simulink model "FBsimDC"  (R2018b)
settings: Solver=ode4  StartTime=0.0  StopTime=0.5e-3*1+0.05*0  FixedStep=Tsim  MaxStep=1e-4  RelTol=1e-6
undefined symbols (not defined in the file): fsw, J, Kt, La, Ra, sigbuilder_block, Ts, Vdc
libraries: powerlib x9, simulink x4, powerlib_meascontrol x1
settings Model: Creator=Mattia  LastModifiedBy=matti
settings DataIOCC: ReturnWorkspaceOutputs=on

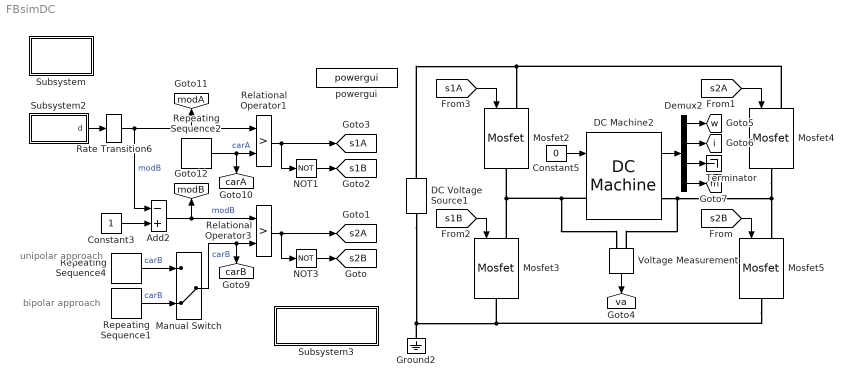
== system FBsimDC ==
  note: unipolar approach
  note: bipolar approach
  Add2 : Sum  Inputs=-+
  Constant3 : Constant  SampleTime=1/(200*fsw)*0+Ts
  Constant5 : Constant  Value=0  SampleTime=1/(200*fsw)
  DC Machine2 : powerlib/Machines/DC Machine  PresetModel=No  MechanicalLoad=Torque TL  FieldType=Permanent magnet  ShowDetailedParameters=on  MeasurementBus=off  RLa="[Ra  La]"  RLf="[ 240  120]"  Laf=1.8  MachineConstant=Torque constant (N.m/A)  Ke=1.8  Kt=Kt  J=J  Bm=B  Tf=0  w0=0  Ifinit=1  TsPowergui=0  TsBlock=-1
      settings: SourceProductName=Simscape Electrical
  DC Voltage Source1 : powerlib/Electrical Sources/DC Voltage Source  Amplitude=Vdc  Measurements=None
      settings: SourceProductName=Simscape Electrical
  Demux2 : Demux  BusSelectionMode=on
  Ground2 : powerlib/Elements/Ground  LConnTagsString=a
      settings: SourceProductName=Simscape Electrical
  Manual Switch : ManualSwitch  CurrentSetting=0
  Mosfet{2..5} (4 alike) : powerlib/Power Electronics/Mosfet  Ron=0.1  Lon=0  Rd=0.01  Vfd=0  IC=0  Rs=1e5  Cs=inf  Measurements=off
      settings: SourceProductName=Simscape Electrical
  NOT1 : Logic  Operator=NOT  IconShape=distinctive  AllPortsSameDT=off  OutDataTypeStr=boolean
  NOT3 : Logic  Operator=NOT  IconShape=distinctive  AllPortsSameDT=off  OutDataTypeStr=boolean
  Rate Transition6 : RateTransition  OutPortSampleTime=Ts
  Relational Operator1 : RelationalOperator  Operator=>  OutDataTypeStr=boolean  RndMeth=Simplest
  Relational Operator3 : RelationalOperator  Operator=>  OutDataTypeStr=boolean  RndMeth=Simplest
  Repeating Sequence1 : simulink/Sources/Repeating Sequence  rep_seq_t=[0 1/(2*fsw) 1/fsw]  rep_seq_y=[1 0 1]
  Repeating Sequence2 : simulink/Sources/Repeating Sequence  rep_seq_t=[0 1/(2*fsw) 1/fsw]  rep_seq_y=[0 1 0]
  Repeating Sequence4 : simulink/Sources/Repeating Sequence  rep_seq_t=[0 1/(2*fsw) 1/fsw]  rep_seq_y=[0 1 0]
  Subsystem : Subsystem
      mask Display: disp('stream')
  Subsystem2 : Subsystem
      mask Display: disp('reference')
  Subsystem3 : Subsystem
      mask Display: disp('embedded version')
  Terminator : Terminator
  Voltage Measurement : powerlib/Measurements/Voltage Measurement  PhasorSimulation=off  OutputType=Complex  PSBequivalent=0
  powergui : powerlib/powergui  Priority=1  SimulationMode=Continuous  SampleTime=1/(400*fsw)  frequency=60  Iterations=50  frequencyindice=0  Pbase=100e6  ErrMax=1e-4  UnitsV=kV  UnitsW=MW  buscounter=0  FunctionMessages=off  echomessages=off  EnableUseOfTLC=off  CurrentSourceSwitches=off  DisableSnubberDevices=on  DisableRonSwitches=on  DisableVfSwitches=on  DisplayEquations=off  SolverType=Tustin/Backward Euler (TBE)  Interpol=off  ExternalGateDelay=off  methode=off  Ts=100  x0status=blocks  SPID=off  SwTol=0  HookPort=off  RestoreLinks=warning  ResistiveCurrentMeasurement=off  Frange=[0:2:500]  Ylog=off  Xlog=on  ShowGrid=off  save=off  variable=ZData  structure=0  ZoomFFT=off  StartTime=0.0  cycles=1  DisplayStyle=1  fundamental=60  FreqAxis=off  MaxFrequency=1000  frequencyindicesteady=1  RmsSteady=1  display=off
  tag scope: carA=global, carB=global, i=global, m=global, modA=global, modB=global, s1A=global, s1B=global, s2A=global, s2B=global, va=global, w=global
  wires:
  NOT1/1 -> [s1B]
  DC Machine2/1 -> Demux2/1
  [s2B] -> Mosfet5/1
  [s2A] -> Mosfet4/1
  [s1B] -> Mosfet3/1
  [s1A] -> Mosfet2/1
  Demux2/3 -> Terminator/1
  Voltage Measurement/1 -> [va]
  Manual Switch/1 -> [carB], Relational Operator3/2  "carB"
  NOT3/1 -> [s2B]
  Repeating Sequence2/1 -> [carA], Relational Operator1/2  "carA"
  Subsystem2/1(d) -> Rate Transition6/1
  Constant3/1 -> Add2/2
  Repeating Sequence4/1 -> Manual Switch/1  "carB"
  Rate Transition6/1 -> Add2/1, Relational Operator1/1, [modA]  "modB"
  Repeating Sequence1/1 -> Manual Switch/2  "carB"
  Constant5/1 -> DC Machine2/1
  Demux2/1 -> [w]
  Demux2/2 -> [i]
  Demux2/4 -> [m]
  Add2/1 -> [modB], Relational Operator3/1  "modB"
  Relational Operator3/1 -> [s2A], NOT3/1
  Relational Operator1/1 -> NOT1/1, [s1A]
  connections:
  Mosfet3/RConn1 -- Mosfet5/RConn1 -- Ground2/LConn1 -- DC Voltage Source1/LConn1
  Mosfet4/LConn1 -- DC Voltage Source1/RConn1 -- Mosfet2/LConn1
  Mosfet4/RConn1 -- Voltage Measurement/LConn2 -- DC Machine2/RConn1 -- Mosfet5/LConn1
  Mosfet3/LConn1 -- Voltage Measurement/LConn1 -- DC Machine2/LConn1 -- Mosfet2/RConn1

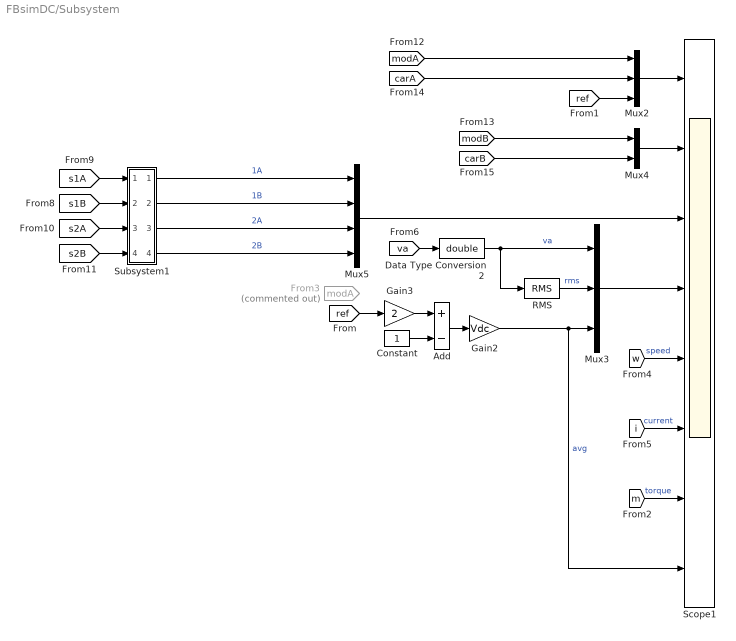
== system FBsimDC/Subsystem ==
  Add : Sum  Inputs=+-
  Constant : Constant  SampleTime=1/(200*fsw)
  Data Type Conversion2 : DataTypeConversion  OutDataTypeStr=double
  From3 : From  Commented=on  GotoTag=modA  TagVisibility=global
  Gain2 : Gain  Gain=Vdc
  Gain3 : Gain  Gain=2
  Mux2 : Mux  Inputs=3
  Mux3 : Mux  Inputs=3
  Mux4 : Mux  Inputs=2
  Mux5 : Mux
  RMS : powerlib_meascontrol/Measurements/RMS  TrueRMS=on  Freq=fsw  RMSInit=0  Ts=0
  Scope1 : Scope  NumInputPorts=8
  Subsystem1 : Subsystem
      mask Display: disp('shift')
  wires:
  Mux3/1 -> Scope1/4
  [s2B] -> Subsystem1/4(In4)
  [s1A] -> Subsystem1/1(In1)
  [va] -> Data Type Conversion2/1
  Mux2/1 -> Scope1/1
  [s2A] -> Subsystem1/3(In3)
  Mux4/1 -> Scope1/2
  [modB] -> Mux4/1
  Data Type Conversion2/1 -> Mux3/1, RMS/1  "va"
  [s1B] -> Subsystem1/2(In2)
  [carB] -> Mux4/2
  Subsystem1/3(Out3) -> Mux5/3  "2A"
  Subsystem1/4(Out4) -> Mux5/4  "2B"
  Subsystem1/2(Out2) -> Mux5/2  "1B"
  Subsystem1/1(Out1) -> Mux5/1  "1A"
  Mux5/1 -> Scope1/3
  [w] -> Scope1/5  "speed"
  [i] -> Scope1/6  "current"
  [m] -> Scope1/7  "torque"
  Gain3/1 -> Add/1
  Gain2/1 -> Mux3/3, Scope1/8  "avg"
  Constant/1 -> Add/2
  [ref] -> Gain3/1
  Add/1 -> Gain2/1
  RMS/1 -> Mux3/2  "rms"
  [carA] -> Mux2/2
  [modA] -> Mux2/1
  [ref] -> Mux2/3

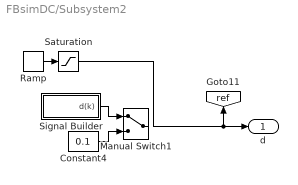
== system FBsimDC/Subsystem2 ==
  Constant4 : Constant  Value=0.1  SampleTime=1/(200*fsw)
  Manual Switch1 : ManualSwitch
  Ramp : simulink/Sources/Ramp  slope=0.9/3e-4  start=0  InitialOutput=0
  Saturation : Saturate  UpperLimit=0.9  LowerLimit=0
  Signal Builder : Subsystem  Tag=STV Subsys  LoadFcn=sigbuilder_block('load');  StartFcn=sigbuilder_block('start');  StopFcn=sigbuilder_block('stop');  ClipboardFcn=sigbuilder_block('clipboard');  mask(Sigbuilder block){tuvar=[0:10]}
      mask help: Simulink:masks:SigbuilderBlock_MD
      mask init:
      | if ~strcmp(get_param(bdroot(gcbh),'SimulationStatus'),'stopped') tuvar = sigbuilder_block('maskInit'); end
      settings: CopyFcn=sigbuilder_block('copy');  DeleteFcn=sigbuilder_block('delete');  ModelCloseFcn=sigbuilder_block('modelClose');  PreSaveFcn=sigbuilder_block('preSave');  PauseFcn=sigbuilder_block('pause');  ContinueFcn=sigbuilder_block('continue');  NameChangeFcn=sigbuilder_block('namechange');  OpenFcn=sigbuilder_block('open',[437.6 199.2 550.4 400 ]);  CloseFcn=sigbuilder_block('close');
      mask Display: plot(0, 0, 100, 100,[2, 2, 32, 32, 2], [68, 8, 8, 68, 68],[32, 2], [38, 38], [32, 19, 2],[53, 60, 44], [32, 17, 17, 2],[16, 16, 31, 31]);txt = getActiveGroup(gcbh);text(2, 100, txt,'verticalAlignment', 'top');
  d : Outport
  tag scope: ref=global
  wires:
  Signal Builder/1(d(k)) -> Manual Switch1/1
  Constant4/1 -> Manual Switch1/2
  Saturation/1 -> d/1, [ref]
  Ramp/1 -> Saturation/1

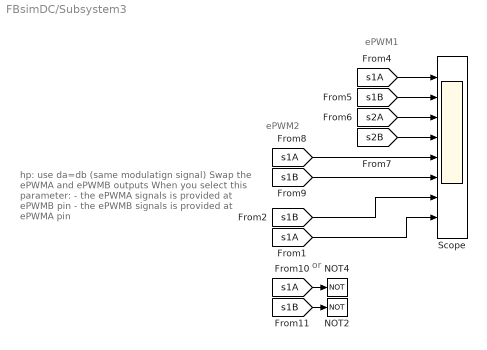
== system FBsimDC/Subsystem3 ==
  note: or
  note: hp: use da=db (same modulatign signal)
      |
      | Swap the ePWMA and ePWMB outputs
      |
      | When you select this parameter:
      | - the ePWMA signals is provided at ePWMB pin
      | - the ePWMB signals is provided at ePWMA pin
  note: ePWM1
  note: ePWM2
  NOT2 : Logic  Operator=NOT  IconShape=distinctive  AllPortsSameDT=off  OutDataTypeStr=boolean
  NOT4 : Logic  Operator=NOT  IconShape=distinctive  AllPortsSameDT=off  OutDataTypeStr=boolean
  Scope : Scope  NumInputPorts=8
  wires:
  [s1A] -> NOT4/1
  [s1B] -> Scope/7
  [s1A] -> Scope/5
  [s2A] -> Scope/3
  [s2B] -> Scope/4
  [s1B] -> Scope/6
  [s1A] -> Scope/8
  [s1B] -> Scope/2
  [s1B] -> NOT2/1
  [s1A] -> Scope/1

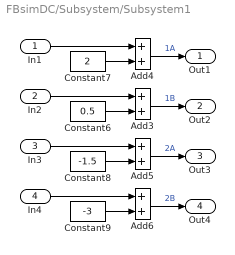
== system FBsimDC/Subsystem/Subsystem1 ==
  In1 : Inport
  In2 : Inport  Port=2
  In3 : Inport  Port=3
  In4 : Inport  Port=4
  Add{3..6} (4 alike) : Sum
  Constant6 : Constant  Value=0.5  SampleTime=1/(200*fsw)*0+Ts
  Constant7 : Constant  Value=2  SampleTime=1/(200*fsw)*0+Ts
  Constant8 : Constant  Value=-1.5  SampleTime=1/(200*fsw)*0+Ts
  Constant9 : Constant  Value=-3  SampleTime=1/(200*fsw)*0+Ts
  Out1 : Outport
  Out2 : Outport  Port=2
  Out3 : Outport  Port=3
  Out4 : Outport  Port=4
  wires:
  In4/1 -> Add6/1
  In2/1 -> Add3/1
  Constant9/1 -> Add6/2
  In1/1 -> Add4/1
  Constant6/1 -> Add3/2
  Constant8/1 -> Add5/2
  Constant7/1 -> Add4/2
  In3/1 -> Add5/1
  Add4/1 -> Out1/1  "1A"
  Add3/1 -> Out2/1  "1B"
  Add5/1 -> Out3/1  "2A"
  Add6/1 -> Out4/1  "2B"

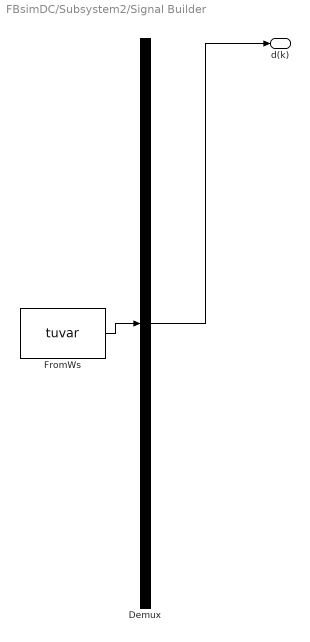
== system FBsimDC/Subsystem2/Signal Builder ==
  Demux : Demux  Tag=STV Demux  Outputs=1
  FromWs : FromWorkspace  Tag=STV FromWs  VariableName=tuvar  SampleTime=0
      SigBuilderData=|
      | common.afterFinalStr = 'Extrapolate'
      | common.sampleTime = 0
      | dataSet.timeRange = [0 0.07]
      | dataSet.name = '  '
      | sbobj.Groups.Name = '  '
      | sbobj.Groups.Signals.Name = 'd(k)'
      | sbobj.Groups.Signals.XData = [0 0.02 0.035 0.045 0.06 0.07]
      | sbobj.Groups.Signals.YData = [0.5 0.9 0.9 0.05 0.05 0]
      | sbobj.Groups.TimeRange = [0 0.07]
  d(k) : Outport  Tag=STV Outport
  wires:
  Demux/1 -> d(k)/1
  FromWs/1 -> Demux/1
